simulink library "speedgoatlib_IO601"  (Simulink 7.3)
settings: Solver=ode45  StartTime=0.0  StopTime=10.0  RelTol=1e-3
undefined symbols (not defined in the file): a, b, sg_init_modules, sg_IO601_cread_m, sg_IO601_linmasterread_m, sg_IO601_linmasterwrite_m, sg_IO601_linslaveread_m, sg_IO601_linslavewrite_m, sg_IO601_read_m, sg_IO601_receive_m, sg_IO601_send_m, sg_IO601_setup_m, sg_IO601_setuplin_m, sg_IO601_status_m, sg_IO601_statuslin_m, sg_IO601_write_m
libraries: simulink x16, xpclib x1, speedgoatlib_IO601 x1
Description:
  | 7.14.0.739 (R2012a)
settings Model: ForwardingTableString=||__slOldName__||speedgoatlib_IO601/Setup||__slNewName__||speedgoatlib_IO601/Obsolete/Setup||__slOldName__||speedgoatlib_IO601/Read status CAN port||__slNewName__||speedgoatlib_IO601/Obsolete/Read status CAN port||__slOldName__||speedgoatlib_IO601/Read||__slNewName__||speedgoatlib_IO601/Obsolete/Read (v2)||__slOldName__||speedgoatlib_IO601/Combined read||__slNewName__||speedgoatlib_IO601/Obsolete/Combined read||__slOldName__||speedgoatlib_IO601/Write||__slNewName__||speedgoatlib_IO601/Obsolete/Write (v2)||__slOldName__||speedgoatlib_IO601/Send||__slNewName__||speedgoatlib_IO601/Obsolete/Send||__slOldName__||speedgoatlib_IO601/Receive||__slNewName__||speedgoatlib_IO601/Obsolete/Receive  Creator=dkuratli  LastModifiedBy=lab3

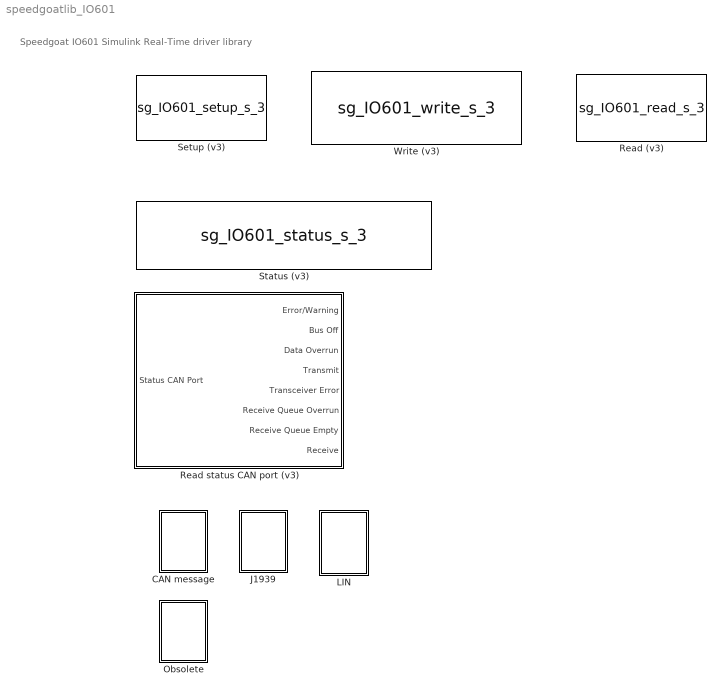
== system speedgoatlib_IO601 ==
  note: Speedgoat IO601 Simulink Real-Time driver library
  CAN message : Subsystem
      settings: OpenFcn=canmsglib
  J1939 : Subsystem
      settings: OpenFcn=xpcJ1939lib
  LIN : Subsystem
  Obsolete : Subsystem
  Read (v3) : S-Function  InitFcn=sg_init_modules('IO601', false, 'setup_IO601_3');  FunctionName=sg_IO601_read_s_3  Parameters=depth1, depth2, outputFormat, port1, port2, sampletime, pciSlot  EnableBusSupport=off  mask(read_IO601_3){id=1, outputFormat=Matrix of doubles (legacy), port1=on, port2=on, depth1=4, depth2=4, sampletime=0.001, pciSlot=-1}
      mask prompts: id "IO601 module identifier:"; outputFormat "Output port datatype:"; port1 "Show CAN message output port 1"; port2 "Show CAN message output port 2"; depth1 "Receive queue read depth:"; depth2 "Receive queue read depth:"; sampletime "Sample time:"; pciSlot "PCI slot (-1: autosearch):"
      mask help: Speedgoat driver block<br>IO601 - Read<br><br>&copy; 2006 - 2014, Speedgoat GmbH, www.speedgoat.ch
      mask init:
      | sg_IO601_read_m_3(id, port1, port2);
      mask Help: web(['C:\Users\lab3\Documents\MATLAB\trunk\thirdpartydrivers\sg_help\comms\dialog_fields_io601_read.htm'],'-helpbrowser');
      mask StyleString: popup(1|2|3|4|5|6|7|8|9|10),popup(Matrix of doubles (legacy)|Vector of CAN_MESSAGE),checkbox,checkbox,edit,edit,edit,edit
      mask TabNameString: Module setup,Input and output port configuration,Input and output port configuration,Input and output port configuration,CAN port 1,CAN port 2,Module setup,Module setup
      mask Display: disp('Speedgoat\nIO601\nRead\nModule: 1');port_label('output', 1, 'CAN port 1');port_label('output', 2, 'count 1');port_label('output', 3, 'CAN port 2');port_label('output', 4, 'count 2');
  Read status CAN port (v3) : Subsystem
      mask Type: readstatuscanport_IO601
      mask Description: This block accepts as an input the output of a CAN Port Status signal from the Read status block and outputs 8 individual status signals.  This block is just a graphical subsystem.
      mask Help: web(fullfile(speedgoatroot,'sg_help','comms','read_status_can_port_driver_block_io601.htm'), '-helpbrowser');
  Setup (v3) : S-Function  InitFcn=sg_init_modules('IO601', true, '');  FunctionName=sg_IO601_setup_s_3  Parameters=can1enable, can1bus, can1UserBR, stdAcc1, extAcc1, can2enable, can2bus, can2UserBR, stdAcc2, extAcc2, pciSlot  EnableBusSupport=off  mask(setup_IO601_3){id=1, can1enable=on, can1bus=Highspeed, can1Baudrate=1 MBaud, can1UserBR=[1,1,5,2], stdAcc1=[0,0,0,0], extAcc1=[0,0,0,0], can2enable=on, can2bus=Highspeed, can2Baudrate=1 MBaud, can2UserBR=[1,1,5,2], stdAcc2=[0,0,0,0], extAcc2=[0,0,0,0], pciSlot=-1}
      mask prompts: id "IO601 module identifier:"; can1enable "Enable"; can1bus "Physical bus:"; can1Baudrate "Baud rate:"; can1UserBR "User defined baud rate [BRP, SJW, TSEG1, TSEG2]:"; stdAcc1 "Acceptance [StdMask1, StdCode1,StdMask2, StdCode2]:"; extAcc1 "Acceptance [ExtMask1, ExtCode1, ExtMask2, ExtCode2]:"; can2enable "Enable"; can2bus "Physical bus:"; can2Baudrate "Baud rate:"; can2UserBR "User defined baud rate [BRP, SJW, TSEG1, TSEG2]:"; stdAcc2 "Acceptance [StdMask1, StdCode1,StdMask2, StdCode2]:"; extAcc2 "Acceptance [ExtMask1, ExtCode1, ExtMask2, ExtCode2]:"; pciSlot "PCI slot (-1: autosearch):"
      mask help: Speedgoat driver block<br>IO601 - Setup<br><br>&copy; 2006 - 2014, Speedgoat GmbH, www.speedgoat.ch
      mask init:
      | can1str='';can2str='';
      | if can1bus==2, can1str=' LS'; end;if can2bus==2, can2str=' LS'; end;
      | %[can1UserBR, can2UserBR, initarray, termarray]= sg_IO601_setup_m(3, id, can1bus, can1Baudrate, can1UserBR, acc1, filter1std, ...
      | %                filter1ext, can2bus, can2Baudrate, can2UserBR, acc2, filter2std, filter2ext, ...
      | %                init, term, pciSlot);
      | 
      | 
      | 
      | [can1UserBR, can2UserBR, stdAcc1, stdAcc2, extAcc1, extAcc2]= sg_IO601_setup_m_3(id, can1Baudrate, can1UserBR, can2Baudrate, can2UserBR, pciSlot, stdAcc1, stdAcc2, extAcc1, extAcc2);
      mask Help: web(['C:\Users\lab3\Documents\MATLAB\trunk\thirdpartydrivers\sg_help\comms\dialog_fields_io601.htm'],'-helpbrowser');
      mask StyleString: popup(1|2|3|4|5|6|7|8|9|10),checkbox,popup(Highspeed |Lowspeed),popup(1 MBaud|800 kBaud|500 kBaud|250 kBaud|125 kBaud|100 kBaud|10 kBaud|User defined),edit,edit,edit,checkbox,popup(Highspeed|Lowspeed),popup(1 MBaud|800 kBaud|500 kBaud|250 kBaud|125 kBaud|100 kBaud|10 kBaud|User defined),edit,edit,edit,edit
      mask TabNameString: Module setup,CAN port 1,CAN port 1,CAN port 1,CAN port 1,CAN port 1,CAN port 1,CAN port 2,CAN port 2,CAN port 2,CAN port 2,CAN port 2,CAN port 2,Module setup
      mask Display: disp('Speedgoat\nIO601\nSetup\nModule: 1');
  Status (v3) : S-Function  InitFcn=sg_init_modules('IO601', false, 'setup_IO601_3');  FunctionName=sg_IO601_status_s_3  Parameters=ts, pciSlot  EnableBusSupport=off  mask(status_IO601_3){id=1, ts=0.001, pciSlot=-1}
      mask prompts: id "IO601 module identifier:"; ts "Sample time:"; pciSlot "PCI slot (-1: autosearch):"
      mask help: Speedgoat driver block<br>IO601 - Status<br><br>&copy; 2006 - 2014, Speedgoat GmbH, www.speedgoat.ch
      mask init:
      | sg_IO601_status_m_3(id)
      mask Help: web(['C:\Users\lab3\Documents\MATLAB\trunk\thirdpartydrivers\sg_help\comms\dialog_fields_io601_status.htm'],'-helpbrowser');
      mask StyleString: popup(1|2|3|4|5|6|7|8|9|10),edit,edit
      mask Display: disp('Speedgoat\nIO601\nStatus\nModule: 1');port_label('output', 1, 'CAN port 1 status');port_label('output', 2, 'CAN port 1 bus last');port_label('output', 3, 'CAN port 2 status');port_label('output', 4, 'CAN port 2 bus last');port_label('output', 5, 'CPU last');port_label('output', 6, 'Live counter');
  Write (v3) : S-Function  Priority=1  InitFcn=sg_init_modules('IO601', false, 'setup_IO601_3');  FunctionName=sg_IO601_write_s_3  Parameters=id, status, inputType, maxMsg, port, initarray, termarray, sampletime, pciSlot  EnableBusSupport=off  mask(write_IO601_3){id=1, sampletime=0.001, pciSlot=-1, inputType=CAN_MESSAGE plus count, port=1, maxMsg=1, status=off, init=[], term=[]}
      mask prompts: id "IO601 module identifier:"; sampletime "Sample time:"; pciSlot "PCI slot (-1: autosearch):"; inputType "CAN message input port datatype:"; port "Port (if input is CAN_MESSAGE):"; maxMsg "CAN messages pool size (only relevant with CAN_MESSAGE option):"; status "Show status output port"; init "Initialization command structure:"; term "Termination command structure:"
      mask help: Speedgoat driver block<br>IO601 - Write<br><br>&copy; 2006 - 2014, Speedgoat GmbH, www.speedgoat.ch
      mask init:
      | [initarray, termarray] = sg_IO601_write_m_3(id, inputType, status, init, term);
      mask Help: web(['C:\Users\lab3\Documents\MATLAB\trunk\thirdpartydrivers\sg_help\comms\dialog_fields_write_io601.htm'],'-helpbrowser');
      mask StyleString: popup(1|2|3|4|5|6|7|8|9|10),edit,edit,popup(Matrix of double (m*5 or m*6)|CAN_MESSAGE plus count),popup(1|2),edit,checkbox,edit,edit
      mask TabNameString: Module setup,Module setup,Module setup,Input and output port configuration,Input and output port configuration,Input and output port configuration,Input and output port configuration,Init and termination setup,Init and termination setup
      mask Display: disp('Speedgoat\nIO601\nWrite\nModule: 1');port_label('input', 1, 'CAN message');port_label('input', 2, 'count');

== system speedgoatlib_IO601/CAN message ==

== system speedgoatlib_IO601/J1939 ==

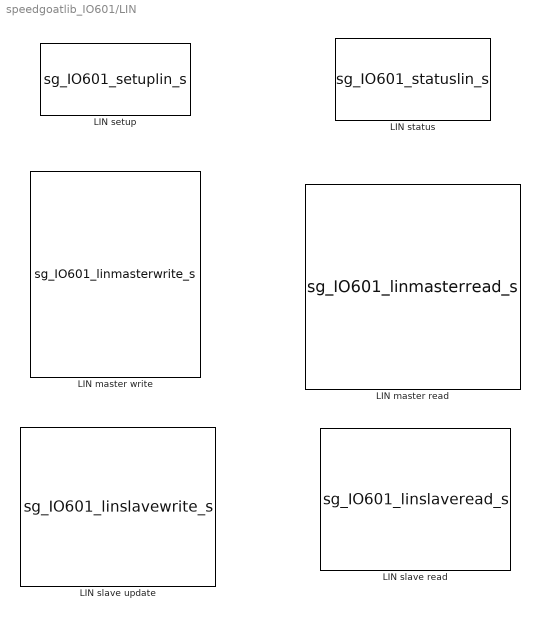
== system speedgoatlib_IO601/LIN ==
  LIN master read : S-Function  InitFcn=sg_IO601_linmasterread_m(1);  FunctionName=sg_IO601_linmasterread_s  Parameters=id, nbMessages, ts, pciSlot  EnableBusSupport=off  mask(masterreadlin_IO601){id=1, nbMessages=1, ts=0.001, pciSlot=-1}
      mask prompts: id "IO601 module identifier:"; nbMessages "Number of messages to read:"; ts "Sample time:"; pciSlot "PCI slot (-1: autosearch):"
      mask help: Speedgoat driver block<br>IO601 - LIN Master read<br><br>&copy; 2006 - 2013, Speedgoat GmbH, www.speedgoat.ch
      mask init:
      | sg_IO601_linmasterread_m(2, id, nbMessages);
      mask Help: Documentation for this block is not available.
      mask StyleString: popup(1|2|3|4|5|6|7|8|9|10),edit,edit,edit
      mask Display: disp('Speedgoat\nIO601\nLIN Master read\nModule: 1');port_label('input',1,'id');port_label('input',2,'length');port_label('output',1,'id');port_label('output',2,'length');port_label('output',3,'data1');port_label('output',4,'data2');port_label('output',5,'data3');port_label('output',6,'data4');port_label('output',7,'data5');port_label('output',8,'data6');port_label('output',9,'data7');port_label('output',10,'data8');port_label('output',11,'timestamp');port_label('output',12,'checksum');port_label('output',13,'type');port_label('output',14,'info');
  LIN master write : S-Function  InitFcn=sg_IO601_linmasterwrite_m(1);  FunctionName=sg_IO601_linmasterwrite_s  Parameters=id, nbMessages, ts, pciSlot  EnableBusSupport=off  mask(masterwritelin_IO601){id=1, nbMessages=1, ts=0.001, pciSlot=-1}
      mask prompts: id "IO601 module identifier:"; nbMessages "Number of messages to write:"; ts "Sample time:"; pciSlot "PCI slot (-1: autosearch):"
      mask help: Speedgoat driver block<br>IO601 - LIN Master write<br><br>&copy; 2006 - 2013, Speedgoat GmbH, www.speedgoat.ch
      mask init:
      | sg_IO601_linmasterwrite_m(2, id, nbMessages);
      mask Help: Documentation for this block is not available.
      mask StyleString: popup(1|2|3|4|5|6|7|8|9|10),edit,edit,edit
      mask Display: disp('Speedgoat\nIO601\nLIN Master write\nModule: 1');port_label('input',1,'type');port_label('input',2,'id');port_label('input',3,'length');port_label('input',4,'data1');port_label('input',5,'data2');port_label('input',6,'data3');port_label('input',7,'data4');port_label('input',8,'data5');port_label('input',9,'data6');port_label('input',10,'data7');port_label('input',11,'data8');
  LIN setup : S-Function  InitFcn=sg_IO601_setuplin_m(1);  FunctionName=sg_IO601_setuplin_s  Parameters=id, baudRate, role, pciSlot  EnableBusSupport=off  mask(setuplin_IO601){id=1, role=Master, baudRate=20000, pciSlot=-1}
      mask prompts: id "IO601 module identifier:"; baudRate "Baudrate (bits/s):"; pciSlot "PCI slot (-1: autosearch):"
      mask help: Speedgoat driver block<br>IO601 - LIN Setup<br><br>&copy; 2006 - 2013, Speedgoat GmbH, www.speedgoat.ch
      mask init:
      | sg_IO601_setuplin_m(2, id, baudRate, pciSlot);
      mask Help: Documentation for this block is not available.
      mask StyleString: popup(1|2|3|4|5|6|7|8|9|10),popup(Slave|Master),edit,edit
      mask Display: disp('Speedgoat\nIO601\nLIN Setup\nModule: 1');
  LIN slave read : S-Function  InitFcn=sg_IO601_linslaveread_m(1);  FunctionName=sg_IO601_linslaveread_s  Parameters=id, nbMessages, ts, pciSlot  EnableBusSupport=off  mask(slavereadlin_IO601){id=1, nbMessages=1, ts=0.001, pciSlot=-1}
      mask prompts: id "IO601 module identifier:"; nbMessages "Number of messages to read:"; ts "Sample time:"; pciSlot "PCI slot (-1: autosearch):"
      mask help: Speedgoat driver block<br>IO601 - LIN Slave read<br><br>&copy; 2006 - 2013, Speedgoat GmbH, www.speedgoat.ch
      mask init:
      | sg_IO601_linslaveread_m(2, id, nbMessages);
      mask Help: Documentation for this block is not available.
      mask StyleString: popup(1|2|3|4|5|6|7|8|9|10),edit,edit,edit
      mask Display: disp('Speedgoat\nIO601\nLIN Slave read\nModule: 1');port_label('output',1,'id');port_label('output',2,'length');port_label('output',3,'data1');port_label('output',4,'data2');port_label('output',5,'data3');port_label('output',6,'data4');port_label('output',7,'data5');port_label('output',8,'data6');port_label('output',9,'data7');port_label('output',10,'data8');port_label('output',11,'timestamp');port_label('output',12,'checksum');port_label('output',13,'type');
  LIN slave update : S-Function  InitFcn=sg_IO601_linslavewrite_m(1);  FunctionName=sg_IO601_linslavewrite_s  Parameters=id, nbMessages, ts, pciSlot  EnableBusSupport=off  mask(slavewritelin_IO601){id=1, nbMessages=1, ts=0.001, pciSlot=-1}
      mask prompts: id "IO601 module identifier:"; nbMessages "Number of messages to update:"; ts "Sample time:"; pciSlot "PCI slot (-1: autosearch):"
      mask help: Speedgoat driver block<br>IO601 - LIN Slave update<br><br>&copy; 2006 - 2013, Speedgoat GmbH, www.speedgoat.ch
      mask init:
      | sg_IO601_linslavewrite_m(2, id, nbMessages);
      mask Help: Documentation for this block is not available.
      mask StyleString: popup(1|2|3|4|5|6|7|8|9|10),edit,edit,edit
      mask Display: disp('Speedgoat\nIO601\nLIN Slave update\nModule: 1');port_label('input',1,'id');port_label('input',2,'length');port_label('input',3,'data1');port_label('input',4,'data2');port_label('input',5,'data3');port_label('input',6,'data4');port_label('input',7,'data5');port_label('input',8,'data6');port_label('input',9,'data7');port_label('input',10,'data8');
  LIN status : S-Function  InitFcn=sg_IO601_statuslin_m(1);  FunctionName=sg_IO601_statuslin_s  Parameters=ts, pciSlot  EnableBusSupport=off  mask(statuslin_IO601){id=1, ts=0.001, pciSlot=[2,4]}
      mask prompts: id "IO601 module identifier:"; ts "Sample time:"; pciSlot "PCI slot (-1: autosearch):"
      mask help: Speedgoat driver block<br>IO601 - LIN Status<br><br>&copy; 2006 - 2013, Speedgoat GmbH, www.speedgoat.ch
      mask init:
      | sg_IO601_statuslin_m(2, id);
      mask Help: Documentation for this block is not available.
      mask StyleString: popup(1|2|3|4|5|6|7|8|9|10),edit,edit
      mask Display: disp('Speedgoat\nIO601\nLIN Status\nModule: 1');port_label('output',1,'role');port_label('output',2,'bus load');port_label('output',3,'baudrate');port_label('output',4,'error flag');

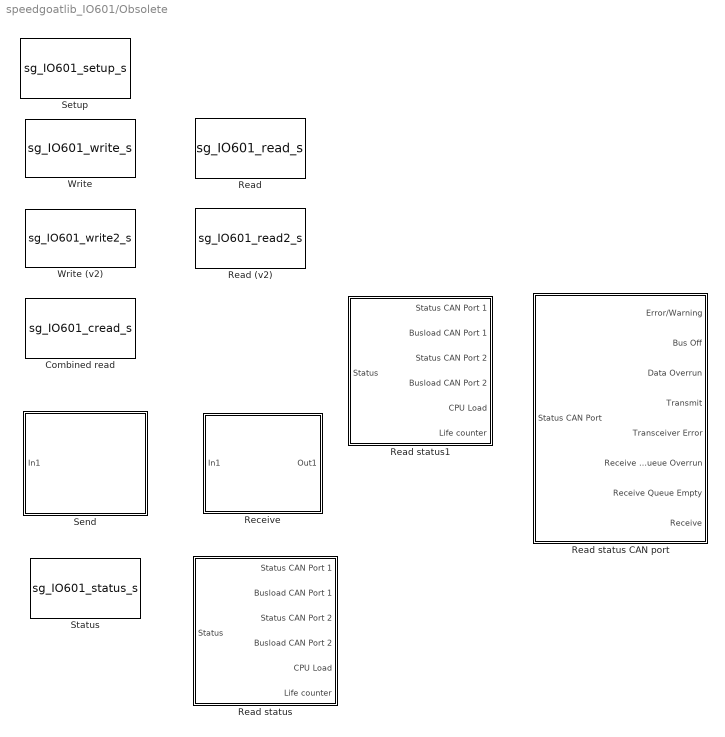
== system speedgoatlib_IO601/Obsolete ==
  Combined read : S-Function  InitFcn=sg_IO601_cread_m(1);  FunctionName=sg_IO601_cread_s  Parameters=id, depth, status, sampletime, pciSlot  EnableBusSupport=off  mask(cread_IO601){id=1, depth=[1,0], status=off, sampletime=0.001, pciSlot=0}
      mask prompts: id "IO601 module identifier:"; depth "Receive queue read depth [CAN port 1, CAN port 2]:"; status "Show status output port"; sampletime "Sample time:"; pciSlot "PCI slot (-1: autosearch):"
      mask help: Speedgoat driver block<br>IO601 - Combined read<br><br>&copy; 2006 - 2013, Speedgoat GmbH, www.speedgoat.ch
      mask init:
      | maskDisplay= sg_IO601_cread_m(2, id);
      mask Help: web(['C:\Program Files\MATLAB\R2013a\toolbox\rtw\targets\xpc\target\build\xpcblocks\thirdpartydrivers\sg_html\io601_combined-read-driver-block.html'],'-helpbrowser');
      mask StyleString: popup(1|2|3|4|5|6|7|8|9|10),edit,checkbox,edit,edit
      mask Display: disp('Speedgoat\nIO601\nCombined read\nModule: 1');
  Read : S-Function  InitFcn=sg_IO601_read_m(1);  FunctionName=sg_IO601_read_s  Parameters=id, port, depth, status, sampletime, pciSlot  EnableBusSupport=off  mask(read_IO601){id=1, port=1, depth=1, status=off, sampletime=0.001, pciSlot=0}
      mask prompts: id "IO601 module identifier:"; port "CAN port:"; depth "Receive queue read depth:"; status "Show status output port"; sampletime "Sample time:"; pciSlot "PCI slot (-1: autosearch):"
      mask help: Speedgoat driver block<br>IO601 - Read<br><br>&copy; 2006 - 2013, Speedgoat GmbH, www.speedgoat.ch
      mask init:
      | maskDisplay= sg_IO601_read_m(2, id);
      mask Help: web(['C:\Program Files\MATLAB\R2013a\toolbox\rtw\targets\xpc\target\build\xpcblocks\thirdpartydrivers\sg_html\io601_read-driver-block-including-can-messaging-support.html'],'-helpbrowser');
      mask StyleString: popup(1|2|3|4|5|6|7|8|9|10),popup(1|2),edit,checkbox,edit,edit
      mask Display: disp('Speedgoat\nIO601\nRead\nModule: 1');
  Read (v2) : S-Function  InitFcn=sg_IO601_read_m(1);  FunctionName=sg_IO601_read2_s  Parameters=id, port, depth, outputFormat, status, sampletime, pciSlot  EnableBusSupport=off  mask(read_IO601){id=1, outputFormat=Vector of CAN_MESSAGE plus count, port=1, depth=1, status=off, sampletime=0.001, pciSlot=-1}
      mask prompts: id "IO601 module identifier:"; outputFormat "Output format:"; port "CAN port:"; depth "Receive queue read depth:"; status "Show status output port"; sampletime "Sample time:"; pciSlot "PCI slot (-1: autosearch):"
      mask help: Speedgoat driver block<br>IO601 - Read<br><br>&copy; 2006 - 2013, Speedgoat GmbH, www.speedgoat.ch
      mask init:
      | maskDisplay= sg_IO601_read_m(2, id);
      mask Help: web(['C:\Program Files\MATLAB\R2013a\toolbox\rtw\targets\xpc\target\build\xpcblocks\thirdpartydrivers\sg_html\io601_read-driver-block-including-can-messaging-support.html'],'-helpbrowser');
      mask StyleString: popup(1|2|3|4|5|6|7|8|9|10),popup(Matrix of doubles (legacy)|Vector of CAN_MESSAGE plus count),popup(1|2),edit,checkbox,edit,edit
      mask Display: disp('Speedgoat\nIO601\nRead\nModule: 1');
  Read status : Subsystem
      mask Type: readstatus_IO601
      mask Description: This block accepts as an input the output of a Status block and outputs the six status elements as individual ports. This block is just a graphical subsystem.
  Read status CAN port : Subsystem
      mask Type: readstatuscanport_IO601
      mask Description: This block accepts as an input the output of a CAN Port Status signal from the Read status block and outputs 8 individual status signals.  This block is just a graphical subsystem.
  Read status1 : Subsystem
      mask Type: readstatus_IO601
      mask Description: This block accepts as an input the output of a Status block and outputs the six status elements as individual ports. This block is just a graphical subsystem.
  Receive : Subsystem  InitFcn=sg_IO601_receive_m(1);  mask(receive_IO601){id=1, canPort=Any, canType=Standard (11-bit), canId=0}
      mask prompts: id "IO601 module identifier:"; canPort "CAN port:"; canType "CAN message type:"; canId "CAN identifier:"
      mask help: Speedgoat driver block<br>IO601 - Receive<br><br>&copy; 2006 - 2013, Speedgoat GmbH, www.speedgoat.ch
      mask init:
      | maskDisplay= sg_IO601_receive_m(2, id, canPort, canType, canId);
      mask Help: Documentation for this block is not available.
      mask StyleString: popup(1|2|3|4|5|6|7|8|9|10),popup(Any|CAN 1|CAN 2),popup(Standard (11-bit)|Extended (29-bit)),edit
      mask Display: disp('Speedgoat\nIO601\nReceive\nModule: 1\nCAN any:  Std\nId: 0 (0x0)');
  Send : Subsystem  InitFcn=sg_IO601_send_m(1);  mask(send_IO601){id=1, canPort=CAN 1, canType=Standard (11-bit), canId=0, canSize=8, ts=0.001}
      mask prompts: id "IO601 module identifier:"; canPort "CAN port:"; canType "CAN message type:"; canId "CAN identifier:"; canSize "CAN data frame size:"; ts "Sample time:"
      mask help: Speedgoat driver block<br>IO601 - Send<br><br>&copy; 2006 - 2013, Speedgoat GmbH, www.speedgoat.ch
      mask init:
      | [a,b,maskDisplay]=sg_IO601_send_m(2, id, canPort, canType, canId, canSize);
      mask Help: Documentation for this block is not available.
      mask StyleString: popup(1|2|3|4|5|6|7|8|9|10),popup(CAN 1|CAN 2),popup(Standard (11-bit)|Extended (29-bit)),edit,edit,edit
      mask Display: disp('Speedgoat\nIO601\nSend\nModule: 1\nCAN 1:  Std, 8\nId: 0 (0x0)');
  Setup : S-Function  InitFcn=sg_IO601_setup_m(1);  FunctionName=sg_IO601_setup_s  Parameters=id, can1enable, can1bus, can1UserBR, acc1, filter1std, filter1ext, can2enable, can2bus, can2UserBR, acc2, filter2std, filter2ext, initarray, termarray, pciSlot  EnableBusSupport=off  mask(setup_IO601){group=Module setup, id=1, can1enable=on, can1bus=Highspeed, can1Baudrate=1 MBaud, can1UserBR=[1,1,5,2], acc1=[0,0,0,0], filter1std=[], filter1ext=[], can2enable=on, can2bus=Highspeed, can2Baudrate=1 MBaud, can2UserBR=[1,1,5,2], acc2=[0,0,0,0], filter2std=[], filter2ext=[], init=[], term=[], pciSlot=-1}
      mask prompts: group "Parameter group:"; id "IO601 module identifier:"; can1enable "Enable"; can1bus "Physical bus:"; can1Baudrate "Baud rate:"; can1UserBR "User defined baud rate [BRP, SJW, TSEG1, TSEG2]:"; acc1 "Acceptance [StdMask, StdCode, ExtMask, ExtCode]:"; filter1std "Standard identifier receive filter vector:"; filter1ext "Extended identifier receive filter vector:"; can2enable "Enable"; can2bus "Physical bus:"; can2Baudrate "Baud rate:"; can2UserBR "User defined baud rate [BRP, SJW, TSEG1, TSEG2]:"; acc2 "Acceptance [StdMask, StdCode, ExtMask, ExtCode]:"; filter2std "Standard identifier receive filter vector:"; filter2ext "Extended identifier receive filter vector:"; init "Initialization command structure:"; term "Termination command structure:"; pciSlot "PCI slot (-1: autosearch):"
      mask help: Speedgoat driver block<br>IO601 - Setup<br><br>&copy; 2006 - 2013, Speedgoat GmbH, www.speedgoat.ch
      mask init:
      | can1str='';can2str='';
      | if can1bus==2, can1str=' LS'; end;if can2bus==2, can2str=' LS'; end;
      | initarray=0;
      | termarray=0;
      | [can1UserBR, can2UserBR, initarray, termarray]= sg_IO601_setup_m(3, id, can1bus, can1Baudrate, can1UserBR, acc1, filter1std, ...
      |                 filter1ext, can2bus, can2Baudrate, can2UserBR, acc2, filter2std, filter2ext, ...
      |                 init, term, pciSlot);
      mask Help: web(['C:\Program Files\MATLAB\R2013a\toolbox\rtw\targets\xpc\target\build\xpcblocks\thirdpartydrivers\sg_html\io601_setup-driver-block.html'],'-helpbrowser');
      mask StyleString: popup(Module setup|CAN 1 port setup|CAN 2 port setup|Initialisation and termination setup),popup(1|2|3|4|5|6|7|8|9|10),checkbox,popup(Highspeed |Lowspeed),popup(1 MBaud|800 kBaud|500 kBaud|250 kBaud|125 kBaud|100 kBaud|10 kBaud|User defined),edit,edit,edit,edit,checkbox,popup(Highspeed|Lowspeed),popup(1 MBaud|800 kBaud|500 kBaud|250 kBaud|125 kBaud|100 kBaud|10 kBaud|User defined),edit,edit,edit,edit,edit,edit,edit
      mask CallbackString: sg_IO601_setup_m(2);||||||||||||||||||
      mask Display: disp('Speedgoat\nIO601\nSetup\nModule: 1');
  Status : S-Function  InitFcn=sg_IO601_status_m(1);  FunctionName=sg_IO601_status_s  Parameters=id, sampletime, pciSlot  EnableBusSupport=off  mask(status_IO601){id=1, sampletime=0.001, pciSlot=0}
      mask prompts: id "IO601 module identifier:"; sampletime "Sample time:"; pciSlot "PCI slot (-1: autosearch):"
      mask help: Speedgoat driver block<br>IO601 - Status<br><br>&copy; 2006 - 2013, Speedgoat GmbH, www.speedgoat.ch
      mask init:
      | maskDisplay= sg_IO601_status_m(2, id);
      mask Help: web(['C:\Program Files\MATLAB\R2013a\toolbox\rtw\targets\xpc\target\build\xpcblocks\thirdpartydrivers\sg_html\io601_status-driver-block.html'],'-helpbrowser');
      mask StyleString: popup(1|2|3|4|5|6|7|8|9|10),edit,edit
      mask Display: disp('Speedgoat\nIO601\nStatus\nModule: 1');
  Write : S-Function  InitFcn=sg_IO601_write_m(1);  FunctionName=sg_IO601_write_s  Parameters=id, status, sampletime, pciSlot  EnableBusSupport=off  mask(write_IO601){id=1, status=off, sampletime=0.001, pciSlot=0}
      mask prompts: id "IO601 module identifier:"; status "Show status output port"; sampletime "Sample time:"; pciSlot "PCI slot (-1: autosearch):"
      mask help: Speedgoat driver block<br>IO601 - Write<br><br>&copy; 2006 - 2013, Speedgoat GmbH, www.speedgoat.ch
      mask init:
      | maskDisplay= sg_IO601_write_m(2, id);
      mask Help: web(['C:\Program Files\MATLAB\R2013a\toolbox\rtw\targets\xpc\target\build\xpcblocks\thirdpartydrivers\sg_html\io601_write-driver-block-including-can-messaging-support.html'],'-helpbrowser');
      mask StyleString: popup(1|2|3|4|5|6|7|8|9|10),checkbox,edit,edit
      mask Display: disp('Speedgoat\nIO601\nWrite\nModule: 1');
  Write (v2) : S-Function  InitFcn=sg_IO601_write_m(1);  FunctionName=sg_IO601_write2_s  Parameters=id, status, inputType, count, maxMsg, port, sampletime, pciSlot  EnableBusSupport=off  mask(write_IO601){id=1, count=on, inputType=CAN_MESSAGE, port=2, maxMsg=20, status=off, sampletime=0.001, pciSlot=-1}
      mask prompts: id "IO601 module identifier:"; count "Show input count port"; inputType "data input port type:"; port "Port (if input is CAN_MESSAGE):"; maxMsg "Max CAN Message Transmit (Per Sample Time):"; status "Show status output port"; sampletime "Sample time:"; pciSlot "PCI slot (-1: autosearch):"
      mask help: Speedgoat driver block<br>IO601 - Write<br><br>&copy; 2006 - 2013, Speedgoat GmbH, www.speedgoat.ch
      mask init:
      | maskDisplay= sg_IO601_write_m(2, id);
      mask Help: web(['C:\Program Files\MATLAB\R2013a\toolbox\rtw\targets\xpc\target\build\xpcblocks\thirdpartydrivers\sg_html\io601_write-driver-block-including-can-messaging-support.html'],'-helpbrowser');
      mask StyleString: popup(1|2|3|4|5|6|7|8|9|10),checkbox,popup(Matrix of double (m*5 or m*6)|CAN_MESSAGE),popup(1|2),edit,checkbox,edit,edit
      mask Display: disp('Speedgoat\nIO601\nWrite\nModule: 1');

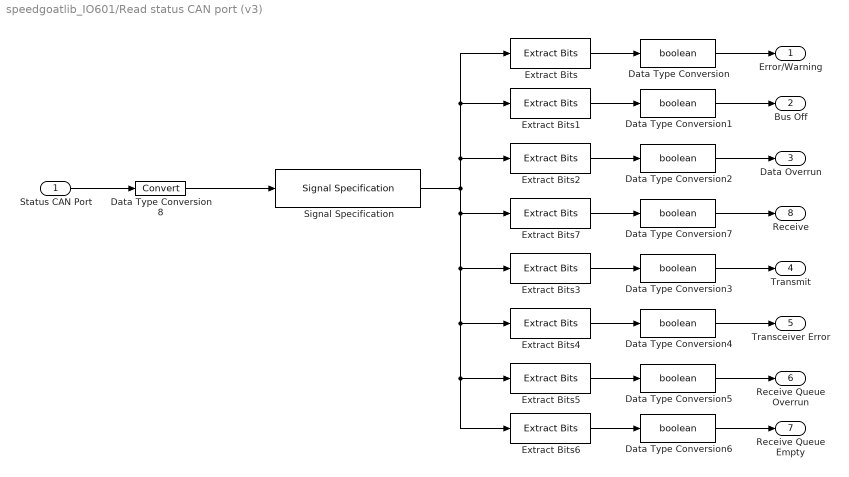
== system speedgoatlib_IO601/Read status CAN port (v3) ==
  Status CAN Port : Inport
  Data Type Conversion{,1..7} (8 alike) : DataTypeConversion  OutDataTypeStr=boolean  OutDataTypeMode=boolean
  Data Type Conversion8 : DataTypeConversion
  Extract Bits : simulink/Logic and Bit Operations/Extract Bits  bitsToExtract=Range of bits  numBits=8  bitIdxRange=[1]  outScalingMode=Preserve fixed-point scaling
  Extract Bits1 : simulink/Logic and Bit Operations/Extract Bits  bitsToExtract=Range of bits  numBits=8  bitIdxRange=[2]  outScalingMode=Preserve fixed-point scaling
  Extract Bits2 : simulink/Logic and Bit Operations/Extract Bits  bitsToExtract=Range of bits  numBits=8  bitIdxRange=[3]  outScalingMode=Preserve fixed-point scaling
  Extract Bits3 : simulink/Logic and Bit Operations/Extract Bits  bitsToExtract=Range of bits  numBits=8  bitIdxRange=[5]  outScalingMode=Preserve fixed-point scaling
  Extract Bits4 : simulink/Logic and Bit Operations/Extract Bits  bitsToExtract=Range of bits  numBits=8  bitIdxRange=[6]  outScalingMode=Preserve fixed-point scaling
  Extract Bits5 : simulink/Logic and Bit Operations/Extract Bits  bitsToExtract=Range of bits  numBits=8  bitIdxRange=[8]  outScalingMode=Preserve fixed-point scaling
  Extract Bits6 : simulink/Logic and Bit Operations/Extract Bits  bitsToExtract=Range of bits  numBits=8  bitIdxRange=[9]  outScalingMode=Preserve fixed-point scaling
  Extract Bits7 : simulink/Logic and Bit Operations/Extract Bits  bitsToExtract=Range of bits  numBits=8  bitIdxRange=[4]  outScalingMode=Preserve fixed-point scaling
  Signal Specification : SignalSpecification  OutDataTypeStr=uint16  Dimensions=1  DataType=uint16
  Error/Warning : Outport
  Bus Off : Outport  Port=2
  Data Overrun : Outport  Port=3
  Transmit : Outport  Port=4
  Transceiver Error : Outport  Port=5
  Receive Queue Overrun : Outport  Port=6
  Receive Queue Empty : Outport  Port=7
  Receive : Outport  Port=8
  wires:
  Data Type Conversion7/1 -> Receive/1
  Extract Bits7/1 -> Data Type Conversion7/1
  Data Type Conversion1/1 -> Bus Off/1
  Data Type Conversion2/1 -> Data Overrun/1
  Data Type Conversion3/1 -> Transmit/1
  Data Type Conversion4/1 -> Transceiver Error/1
  Data Type Conversion5/1 -> Receive Queue Overrun/1
  Data Type Conversion6/1 -> Receive Queue Empty/1
  Extract Bits6/1 -> Data Type Conversion6/1
  Extract Bits5/1 -> Data Type Conversion5/1
  Extract Bits4/1 -> Data Type Conversion4/1
  Extract Bits3/1 -> Data Type Conversion3/1
  Extract Bits2/1 -> Data Type Conversion2/1
  Extract Bits1/1 -> Data Type Conversion1/1
  Data Type Conversion/1 -> Error/Warning/1
  Extract Bits/1 -> Data Type Conversion/1
  Status CAN Port/1 -> Data Type Conversion8/1
  Signal Specification/1 -> Extract Bits7/1, Extract Bits3/1, Extract Bits4/1, Extract Bits5/1, Extract Bits6/1, Extract Bits2/1, Extract Bits1/1, Extract Bits/1
  Data Type Conversion8/1 -> Signal Specification/1

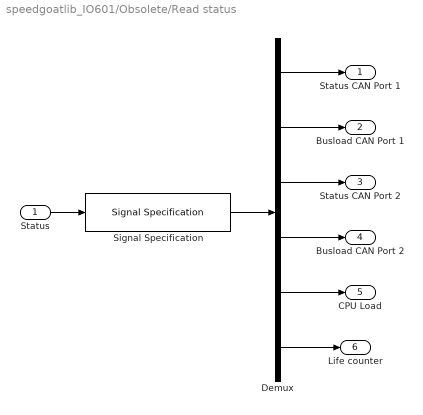
== system speedgoatlib_IO601/Obsolete/Read status ==
  Status : Inport
  Demux : Demux  Outputs=6
  Signal Specification : SignalSpecification  OutDataTypeStr=uint16  Dimensions=6  DataType=uint16
  Status CAN Port 1 : Outport
  Busload CAN Port 1 : Outport  Port=2
  Status CAN Port 2 : Outport  Port=3
  Busload CAN Port 2 : Outport  Port=4
  CPU Load : Outport  Port=5
  Life counter : Outport  Port=6
  wires:
  Signal Specification/1 -> Demux/1
  Demux/1 -> Status CAN Port 1/1
  Demux/2 -> Busload CAN Port 1/1
  Demux/3 -> Status CAN Port 2/1
  Status/1 -> Signal Specification/1
  Demux/4 -> Busload CAN Port 2/1
  Demux/5 -> CPU Load/1
  Demux/6 -> Life counter/1

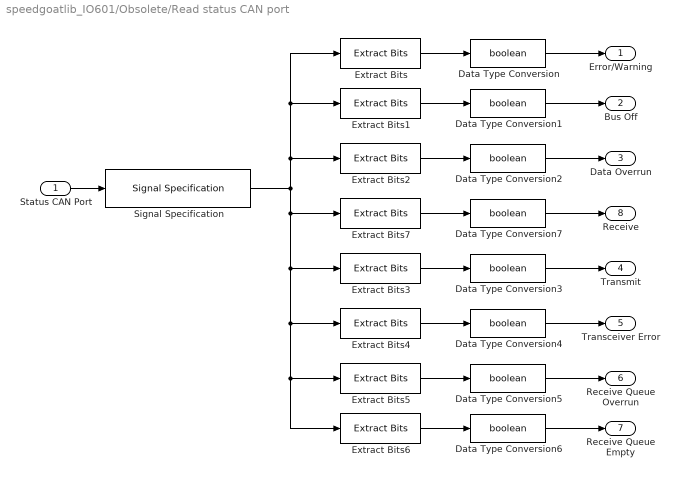
== system speedgoatlib_IO601/Obsolete/Read status CAN port ==
  Status CAN Port : Inport
  Data Type Conversion{,1..7} (8 alike) : DataTypeConversion  OutDataTypeStr=boolean  OutDataTypeMode=boolean
  Extract Bits : simulink/Logic and Bit Operations/Extract Bits  bitsToExtract=Range of bits  numBits=8  bitIdxRange=[1]  outScalingMode=Preserve fixed-point scaling
  Extract Bits1 : simulink/Logic and Bit Operations/Extract Bits  bitsToExtract=Range of bits  numBits=8  bitIdxRange=[2]  outScalingMode=Preserve fixed-point scaling
  Extract Bits2 : simulink/Logic and Bit Operations/Extract Bits  bitsToExtract=Range of bits  numBits=8  bitIdxRange=[3]  outScalingMode=Preserve fixed-point scaling
  Extract Bits3 : simulink/Logic and Bit Operations/Extract Bits  bitsToExtract=Range of bits  numBits=8  bitIdxRange=[5]  outScalingMode=Preserve fixed-point scaling
  Extract Bits4 : simulink/Logic and Bit Operations/Extract Bits  bitsToExtract=Range of bits  numBits=8  bitIdxRange=[6]  outScalingMode=Preserve fixed-point scaling
  Extract Bits5 : simulink/Logic and Bit Operations/Extract Bits  bitsToExtract=Range of bits  numBits=8  bitIdxRange=[8]  outScalingMode=Preserve fixed-point scaling
  Extract Bits6 : simulink/Logic and Bit Operations/Extract Bits  bitsToExtract=Range of bits  numBits=8  bitIdxRange=[9]  outScalingMode=Preserve fixed-point scaling
  Extract Bits7 : simulink/Logic and Bit Operations/Extract Bits  bitsToExtract=Range of bits  numBits=8  bitIdxRange=[4]  outScalingMode=Preserve fixed-point scaling
  Signal Specification : SignalSpecification  OutDataTypeStr=uint16  Dimensions=1  DataType=uint16
  Error/Warning : Outport
  Bus Off : Outport  Port=2
  Data Overrun : Outport  Port=3
  Transmit : Outport  Port=4
  Transceiver Error : Outport  Port=5
  Receive Queue Overrun : Outport  Port=6
  Receive Queue Empty : Outport  Port=7
  Receive : Outport  Port=8
  wires:
  Signal Specification/1 -> Extract Bits/1, Extract Bits1/1, Extract Bits2/1, Extract Bits6/1, Extract Bits5/1, Extract Bits4/1, Extract Bits3/1, Extract Bits7/1
  Status CAN Port/1 -> Signal Specification/1
  Extract Bits/1 -> Data Type Conversion/1
  Data Type Conversion/1 -> Error/Warning/1
  Extract Bits1/1 -> Data Type Conversion1/1
  Extract Bits2/1 -> Data Type Conversion2/1
  Extract Bits3/1 -> Data Type Conversion3/1
  Extract Bits4/1 -> Data Type Conversion4/1
  Extract Bits5/1 -> Data Type Conversion5/1
  Extract Bits6/1 -> Data Type Conversion6/1
  Data Type Conversion6/1 -> Receive Queue Empty/1
  Data Type Conversion5/1 -> Receive Queue Overrun/1
  Data Type Conversion4/1 -> Transceiver Error/1
  Data Type Conversion3/1 -> Transmit/1
  Data Type Conversion2/1 -> Data Overrun/1
  Data Type Conversion1/1 -> Bus Off/1
  Extract Bits7/1 -> Data Type Conversion7/1
  Data Type Conversion7/1 -> Receive/1

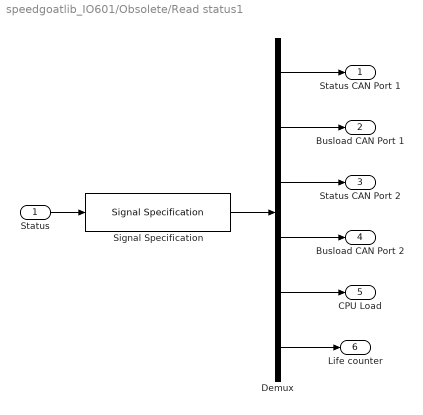
== system speedgoatlib_IO601/Obsolete/Read status1 ==
  Status : Inport
  Demux : Demux  Outputs=6
  Signal Specification : SignalSpecification  OutDataTypeStr=uint16  Dimensions=6  DataType=uint16
  Status CAN Port 1 : Outport
  Busload CAN Port 1 : Outport  Port=2
  Status CAN Port 2 : Outport  Port=3
  Busload CAN Port 2 : Outport  Port=4
  CPU Load : Outport  Port=5
  Life counter : Outport  Port=6
  wires:
  Signal Specification/1 -> Demux/1
  Demux/1 -> Status CAN Port 1/1
  Demux/2 -> Busload CAN Port 1/1
  Demux/3 -> Status CAN Port 2/1
  Status/1 -> Signal Specification/1
  Demux/4 -> Busload CAN Port 2/1
  Demux/5 -> CPU Load/1
  Demux/6 -> Life counter/1

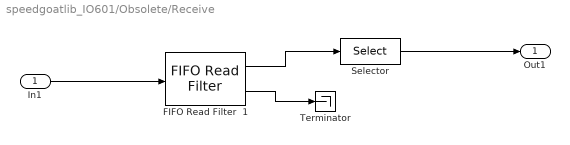
== system speedgoatlib_IO601/Obsolete/Receive ==
  In1 : Inport
  FIFO Read Filter  1 : xpclib/CAN/Softing/CAN-AC2-PCI SJA 1000/FIFO Mode/FIFO Read Filter   portin=Any  ctypein=SDF  direction=Include  ident=canId  identsel=Include
  Selector : Selector  InputPortWidth=6  Indices=[6]
  Terminator : Terminator
  Out1 : Outport
  wires:
  FIFO Read Filter  1/1 -> Selector/1
  FIFO Read Filter  1/2 -> Terminator/1
  In1/1 -> FIFO Read Filter  1/1
  Selector/1 -> Out1/1

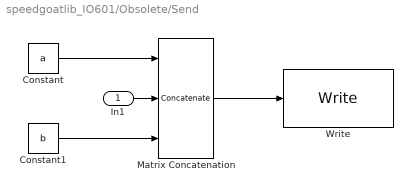
== system speedgoatlib_IO601/Obsolete/Send ==
  In1 : Inport  PortDimensions=1
  Constant : Constant  Value=a  VectorParams1D=off
  Constant1 : Constant  Value=b  VectorParams1D=off
  Matrix Concatenation : Concatenate  NumInputs=3  Mode=Multidimensional array  ConcatenateDimension=2
  Write : speedgoatlib_IO601/Obsolete/Write  id=1  status=off  sampletime=ts  pciSlot=0
  wires:
  Matrix Concatenation/1 -> Write/1
  Constant/1 -> Matrix Concatenation/1
  Constant1/1 -> Matrix Concatenation/3
  In1/1 -> Matrix Concatenation/2
